simulink model "Es34"  (R2021b)
settings: Solver=FixedStepAuto  StartTime=0.0  StopTime=3  FixedStep=1e-3  RelTol=1e-5
undefined symbols (not defined in the file or in its folder): coriolis, epsilon, gravload, inertia, Kd, Kp, p560, p560_nofric, p560Unc, p560Unc_nf, q_init, rho, Z, Z_1, Z_10
libraries: simulink x5
settings Model: Creator=Andrea  LastModifiedBy=mular
settings SolverCC: AlgebraicLoopSolver=TrustRegion
settings DataIOCC: ReturnWorkspaceOutputs=off
settings DebuggingCC: SFMachineParentedDataDiag=warning  ArithmeticOperatorsInVariantConditions=warning
settings SFSimCC: CustomCodeUndefinedFunction=UseInterfaceOnly

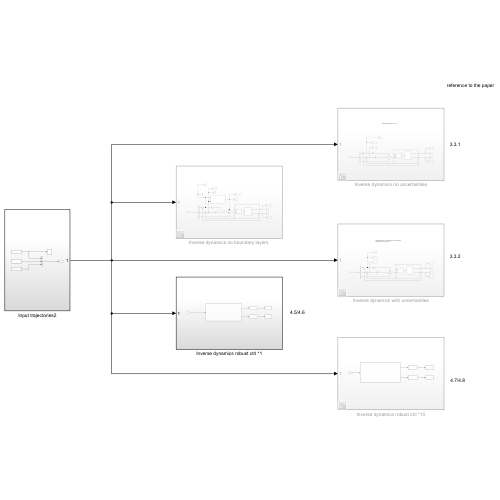
[thumbnail: Simulink's stored preview of the top-level diagram]
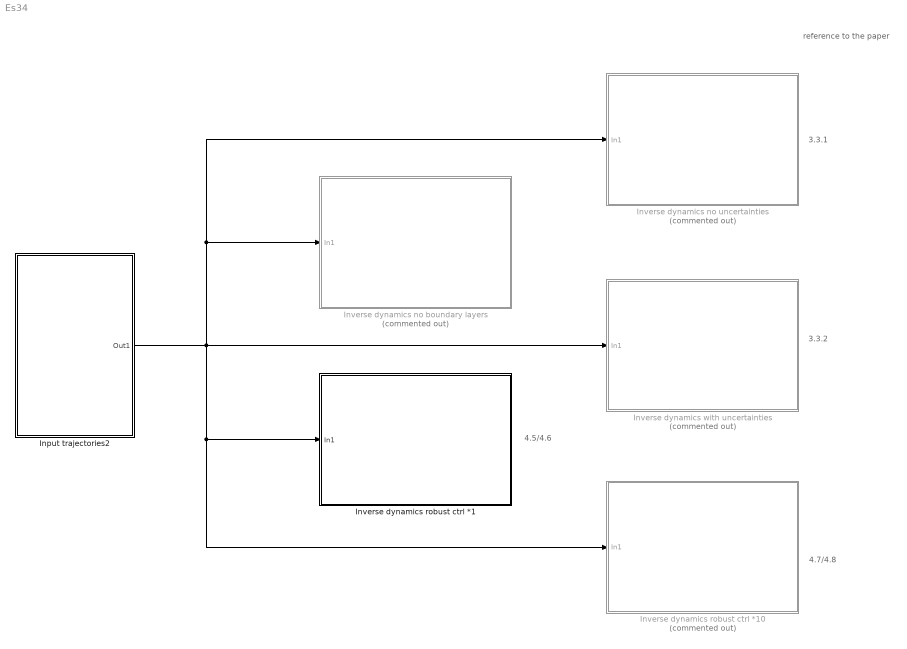
== system Es34 ==
  note: reference to the paper
  note: 4.5/4.6
  note: 4.7/4.8
  note: 3.3.2
  note: 3.3.1
  Input trajectories2 : Subsystem
  "Inverse dynamics no boundary layers " : Subsystem  Commented=on
  Inverse dynamics no uncertainties : Subsystem  Commented=on
  Inverse dynamics robust ctrl *1 : Subsystem
  Inverse dynamics robust ctrl *10 : Subsystem  Commented=on
  Inverse dynamics with uncertainties : Subsystem  Commented=on
  wires:
  Input trajectories2/1(Out1) -> Inverse dynamics no uncertainties/1(In1), "Inverse dynamics no boundary layers "/1(In1), Inverse dynamics robust ctrl *10/1(In1), Inverse dynamics robust ctrl *1/1(In1), Inverse dynamics with uncertainties/1(In1)

== system Es34/Input trajectories2 ==
  From Workspace : FromWorkspace  VariableName=qqs  OutputAfterFinalValue=Holding final value
  From Workspace1 : FromWorkspace  VariableName=qqsd  OutputAfterFinalValue=Holding final value
  From Workspace2 : FromWorkspace  VariableName=qqsdd  OutputAfterFinalValue=Holding final value
  Mux : Mux  Inputs=3
  Scope : Scope
  Out1 : Outport  VectorParamsAs1DForOutWhenUnconnected=off
  wires:
  Mux/1 -> Out1/1
  From Workspace1/1 -> Mux/2
  From Workspace/1 -> Mux/1, Scope/1
  From Workspace2/1 -> Mux/3

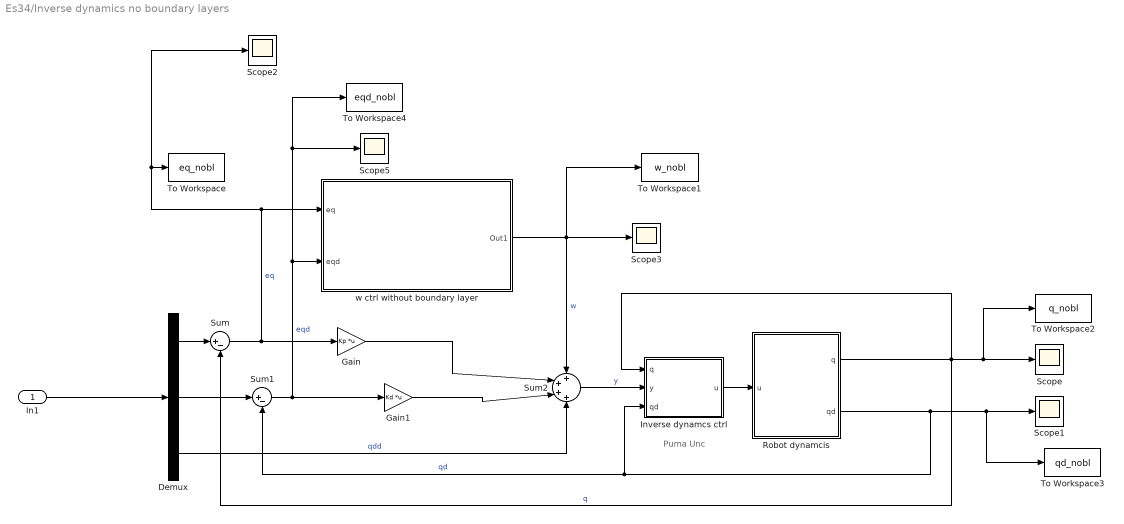
== system Es34/Inverse dynamics no boundary layers  ==
  note: Puma Unc
  In1 : Inport
  Demux : Demux  Outputs=3
  Gain : Gain  Gain=Kp  Multiplication=Matrix(K*u) (u vector)
  Gain1 : Gain  Gain=Kd  Multiplication=Matrix(K*u) (u vector)
  Inverse dynamcs ctrl : Subsystem  mask{mdl=p560Unc}
      mask prompts: mdl "Robot model"
  Robot dynamcis : Subsystem  mask{Realmdl=p560_nofric, q_init=q_init}
      mask prompts: Realmdl "Real robot model"; q_init "Initial position"
  Scope{,1..3,5} (5 alike) : Scope
  Sum : Sum  Inputs=|+-
  Sum1 : Sum  Inputs=|+-
  Sum2 : Sum  Inputs=++++
  To Workspace : ToWorkspace  VariableName=eq_nobl  SampleTime=-1
  To Workspace1 : ToWorkspace  VariableName=w_nobl  SampleTime=-1
  To Workspace2 : ToWorkspace  VariableName=q_nobl  SampleTime=-1
  To Workspace3 : ToWorkspace  VariableName=qd_nobl  SampleTime=-1
  To Workspace4 : ToWorkspace  VariableName=eqd_nobl  SampleTime=-1
  w ctrl without boundary layer : Subsystem
  wires:
  Sum/1 -> Gain/1, w ctrl without boundary layer/1(eq), To Workspace/1, Scope2/1  "eq"
  Sum2/1 -> Inverse dynamcs ctrl/2(y)  "y"
  Sum1/1 -> To Workspace4/1, Scope5/1, w ctrl without boundary layer/2(eqd), Gain1/1  "eqd"
  Demux/2 -> Sum1/1
  Demux/1 -> Sum/1
  Inverse dynamcs ctrl/1(u) -> Robot dynamcis/1(u)
  In1/1 -> Demux/1
  Demux/3 -> Sum2/4  "qdd"
  w ctrl without boundary layer/1(Out1) -> Scope3/1, To Workspace1/1, Sum2/1  "w"
  Robot dynamcis/1(q) -> Inverse dynamcs ctrl/1(q), To Workspace2/1, Scope/1, Sum/2  "q"
  Robot dynamcis/2(qd) -> Scope1/1, To Workspace3/1, Inverse dynamcs ctrl/3(qd), Sum1/2  "qd"
  Gain1/1 -> Sum2/3
  Gain/1 -> Sum2/2

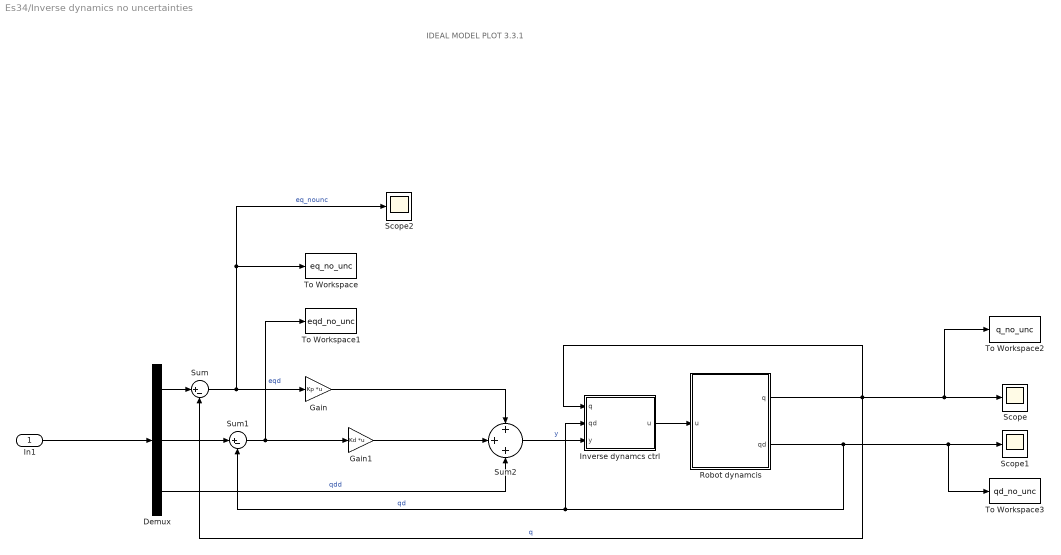
== system Es34/Inverse dynamics no uncertainties ==
  note: IDEAL MODEL PLOT 3.3.1
  In1 : Inport
  Demux : Demux  Outputs=3
  Gain : Gain  Gain=Kp  Multiplication=Matrix(K*u) (u vector)
  Gain1 : Gain  Gain=Kd  Multiplication=Matrix(K*u) (u vector)
  Inverse dynamcs ctrl : Subsystem  mask{mdl=p560Unc_nf}
      mask prompts: mdl "Robot model"
  Robot dynamcis : Subsystem  mask{Realmdl=p560Unc_nf, q_init=q_init}
      mask prompts: Realmdl "Real robot model"; q_init "Initial position"
  Scope : Scope
  Scope1 : Scope
  Scope2 : Scope
  Sum : Sum  Inputs=|+-
  Sum1 : Sum  Inputs=|+-
  Sum2 : Sum  Inputs=+++
  To Workspace : ToWorkspace  VariableName=eq_no_unc  SampleTime=-1
  To Workspace1 : ToWorkspace  VariableName=eqd_no_unc  SampleTime=-1
  To Workspace2 : ToWorkspace  VariableName=q_no_unc  SampleTime=-1
  To Workspace3 : ToWorkspace  VariableName=qd_no_unc  SampleTime=-1
  wires:
  Robot dynamcis/2(qd) -> To Workspace3/1, Scope1/1, Sum1/2, Inverse dynamcs ctrl/2(qd)  "qd"
  Robot dynamcis/1(q) -> Inverse dynamcs ctrl/1(q), To Workspace2/1, Scope/1, Sum/2  "q"
  Gain1/1 -> Sum2/2
  In1/1 -> Demux/1
  Inverse dynamcs ctrl/1(u) -> Robot dynamcis/1(u)
  Demux/1 -> Sum/1
  Demux/2 -> Sum1/1
  Sum1/1 -> To Workspace1/1, Gain1/1  "eqd"
  Sum2/1 -> Inverse dynamcs ctrl/3(y)  "y"
  Sum/1 -> Scope2/1, To Workspace/1, Gain/1  "eq_nounc"
  Gain/1 -> Sum2/1
  Demux/3 -> Sum2/3  "qdd"

== system Es34/Inverse dynamics robust ctrl *1 ==
  In1 : Inport
  Interpreted MATLAB Function1 : MATLABFcn  MATLABFcn=norm(u,2)  OutputDimensions=1
  Interpreted MATLAB Function2 : MATLABFcn  MATLABFcn=norm(u,2)  OutputDimensions=1
  To Workspace : ToWorkspace  VariableName=norm_eq_rc1  SampleTime=-1
  To Workspace1 : ToWorkspace  VariableName=norm_eqd_rc1  SampleTime=-1
  ctrl : Subsystem
  wires:
  In1/1 -> ctrl/1(In1)
  ctrl/1(eq) -> Interpreted MATLAB Function1/1
  Interpreted MATLAB Function1/1 -> To Workspace/1
  Interpreted MATLAB Function2/1 -> To Workspace1/1
  ctrl/2(eqd) -> Interpreted MATLAB Function2/1

== system Es34/Inverse dynamics robust ctrl *10 ==
  In1 : Inport
  Interpreted MATLAB Function1 : MATLABFcn  MATLABFcn=norm(u,2)  OutputDimensions=1
  Interpreted MATLAB Function2 : MATLABFcn  MATLABFcn=norm(u,2)  OutputDimensions=1
  To Workspace : ToWorkspace  VariableName=norm_eq_rc10  SampleTime=-1
  To Workspace1 : ToWorkspace  VariableName=norm_eqd_rc10  SampleTime=-1
  ctrl : Subsystem
  wires:
  ctrl/2(eqd) -> Interpreted MATLAB Function2/1
  Interpreted MATLAB Function2/1 -> To Workspace1/1
  Interpreted MATLAB Function1/1 -> To Workspace/1
  ctrl/1(eq) -> Interpreted MATLAB Function1/1
  In1/1 -> ctrl/1(In1)

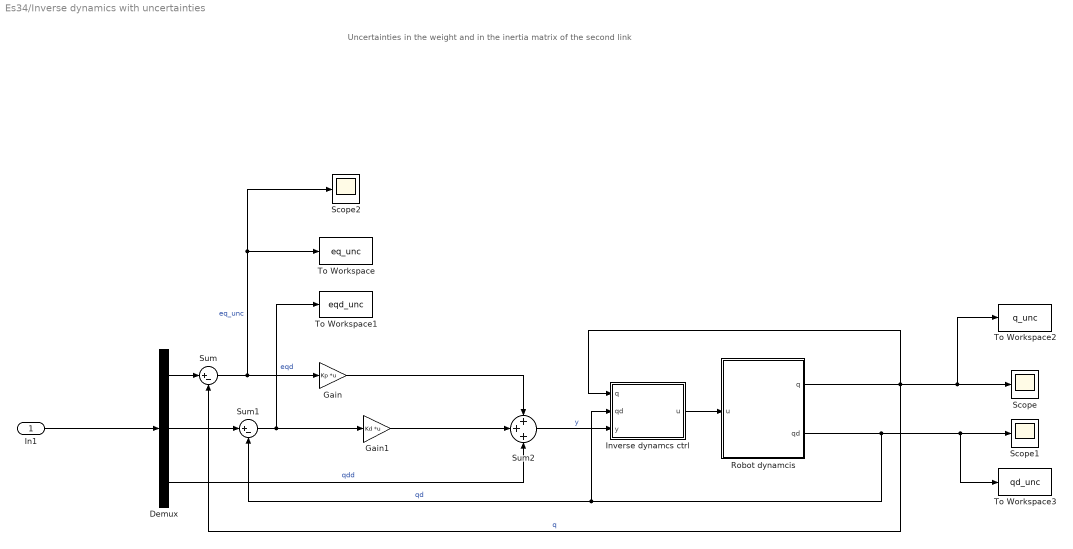
== system Es34/Inverse dynamics with uncertainties ==
  note: Uncertainties in the weight and in the inertia matrix of the second link
  In1 : Inport
  Demux : Demux  Outputs=3
  Gain : Gain  Gain=Kp  Multiplication=Matrix(K*u) (u vector)
  Gain1 : Gain  Gain=Kd  Multiplication=Matrix(K*u) (u vector)
  Inverse dynamcs ctrl : Subsystem  mask{mdl=p560Unc_nf}
      mask prompts: mdl "Robot model"
  Robot dynamcis : Subsystem  mask{Realmdl=p560_nofric, q_init=q_init}
      mask prompts: Realmdl "Real robot model"; q_init "Initial position"
  Scope : Scope
  Scope1 : Scope
  Scope2 : Scope
  Sum : Sum  Inputs=|+-
  Sum1 : Sum  Inputs=|+-
  Sum2 : Sum  Inputs=+++
  To Workspace : ToWorkspace  VariableName=eq_unc  SampleTime=-1
  To Workspace1 : ToWorkspace  VariableName=eqd_unc  SampleTime=-1
  To Workspace2 : ToWorkspace  VariableName=q_unc  SampleTime=-1
  To Workspace3 : ToWorkspace  VariableName=qd_unc  SampleTime=-1
  wires:
  Sum/1 -> Gain/1, Scope2/1, To Workspace/1  "eq_unc"
  Sum2/1 -> Inverse dynamcs ctrl/3(y)  "y"
  Sum1/1 -> To Workspace1/1, Gain1/1  "eqd"
  Demux/2 -> Sum1/1
  Demux/1 -> Sum/1
  Inverse dynamcs ctrl/1(u) -> Robot dynamcis/1(u)
  In1/1 -> Demux/1
  Demux/3 -> Sum2/3  "qdd"
  Gain1/1 -> Sum2/2
  Robot dynamcis/1(q) -> Inverse dynamcs ctrl/1(q), To Workspace2/1, Scope/1, Sum/2  "q"
  Robot dynamcis/2(qd) -> To Workspace3/1, Scope1/1, Inverse dynamcs ctrl/2(qd), Sum1/2  "qd"
  Gain/1 -> Sum2/1

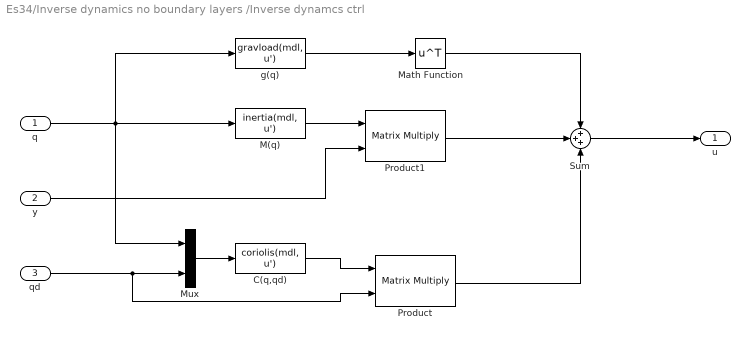
== system Es34/Inverse dynamics no boundary layers /Inverse dynamcs ctrl ==
  q : Inport
  y : Inport  Port=2
  qd : Inport  Port=3
  C(q,qd) : MATLABFcn  MATLABFcn=coriolis(mdl, u')  OutputDimensions=[p560.n p560.n]  Output1D=off
  M(q) : MATLABFcn  MATLABFcn=inertia(mdl, u')  OutputDimensions=[p560.n p560.n]  Output1D=off
  Math Function : Math  Operator=transpose  SignedPower=on  SaturateOnIntegerOverflow=on
  Mux : Mux  Inputs=2
  Product : Product  Multiplication=Matrix(*)
  Product1 : Product  Multiplication=Matrix(*)
  Sum : Sum  Inputs=+++
  g(q) : MATLABFcn  MATLABFcn=gravload(mdl, u')  OutputDimensions=[1 p560.n]  Output1D=off
  u : Outport  VectorParamsAs1DForOutWhenUnconnected=off
  wires:
  q/1 -> M(q)/1, g(q)/1, Mux/1
  Mux/1 -> C(q,qd)/1
  C(q,qd)/1 -> Product/1
  qd/1 -> Product/2, Mux/2
  M(q)/1 -> Product1/1
  y/1 -> Product1/2
  Product1/1 -> Sum/2
  Product/1 -> Sum/3
  Sum/1 -> u/1
  g(q)/1 -> Math Function/1
  Math Function/1 -> Sum/1

== system Es34/Inverse dynamics no boundary layers /Robot dynamcis ==
  u : Inport
  Integrator : Integrator
  Integrator1 : Integrator  InitialCondition=q_init
  Mux : Mux  Inputs=3
  S-Function : S-Function  FunctionName=slaccel  Parameters=Realmdl  SFunctionDeploymentMode=off  EnableBusSupport=off
  q : Outport  VectorParamsAs1DForOutWhenUnconnected=off
  qd : Outport  Port=2  VectorParamsAs1DForOutWhenUnconnected=off
  wires:
  Mux/1 -> S-Function/1
  u/1 -> Mux/3
  Integrator/1 -> qd/1, Mux/2, Integrator1/1  "qd"
  S-Function/1 -> Integrator/1  "qdd"
  Integrator1/1 -> q/1, Mux/1

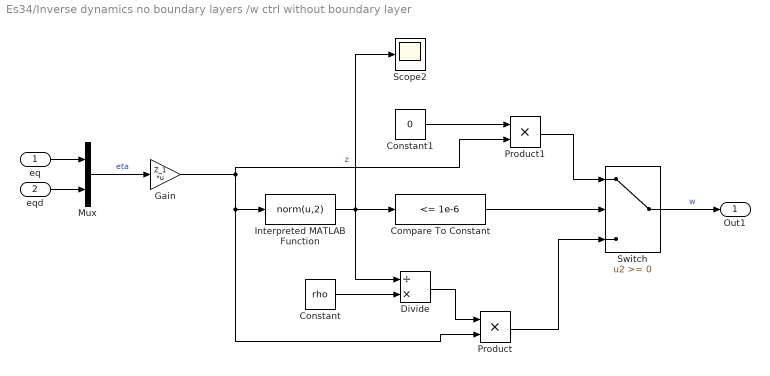
== system Es34/Inverse dynamics no boundary layers /w ctrl without boundary layer ==
  eq : Inport
  eqd : Inport  Port=2
  Compare To Constant : simulink/Logic and Bit Operations/Compare To Constant  relop=<=  const=1e-6  OutDataTypeStr=boolean  ZeroCross=off
  Constant : Constant  Value=rho
  Constant1 : Constant  Value=0
  Divide : Product  Inputs=/*
  Gain : Gain  Gain=Z_1  Multiplication=Matrix(K*u) (u vector)
  Interpreted MATLAB Function : MATLABFcn  MATLABFcn=norm(u,2)
  Mux : Mux  Inputs=2
  Product : Product
  Product1 : Product
  Scope2 : Scope
  Switch : Switch  ZeroCross=off
  Out1 : Outport  VectorParamsAs1DForOutWhenUnconnected=off
  wires:
  eqd/1 -> Mux/2
  Mux/1 -> Gain/1  "eta"
  eq/1 -> Mux/1
  Gain/1 -> Interpreted MATLAB Function/1, Product/2, Product1/2  "z"
  Interpreted MATLAB Function/1 -> Scope2/1, Divide/1, Compare To Constant/1
  Switch/1 -> Out1/1  "w"
  Constant/1 -> Divide/2
  Divide/1 -> Product/1
  Compare To Constant/1 -> Switch/2
  Product/1 -> Switch/3
  Constant1/1 -> Product1/1
  Product1/1 -> Switch/1

== system Es34/Inverse dynamics no uncertainties/Inverse dynamcs ctrl ==
  q : Inport
  qd : Inport  Port=2
  y : Inport  Port=3
  C(q,qd) : MATLABFcn  MATLABFcn=coriolis(mdl, u')  OutputDimensions=[p560.n p560.n]  Output1D=off
  M(q) : MATLABFcn  MATLABFcn=inertia(mdl, u')  OutputDimensions=[p560.n p560.n]  Output1D=off
  Math Function : Math  Operator=transpose  SignedPower=on  SaturateOnIntegerOverflow=on
  Mux : Mux  Inputs=2
  Product : Product  Multiplication=Matrix(*)
  Product1 : Product  Multiplication=Matrix(*)
  Sum : Sum  Inputs=+++
  g(q) : MATLABFcn  MATLABFcn=gravload(mdl, u')  OutputDimensions=[1 p560.n]  Output1D=off
  u : Outport  VectorParamsAs1DForOutWhenUnconnected=off
  wires:
  Math Function/1 -> Sum/1
  g(q)/1 -> Math Function/1
  Sum/1 -> u/1
  Product/1 -> Sum/3
  Product1/1 -> Sum/2
  y/1 -> Product1/2
  M(q)/1 -> Product1/1
  qd/1 -> Mux/2, Product/2
  C(q,qd)/1 -> Product/1
  Mux/1 -> C(q,qd)/1
  q/1 -> Mux/1, M(q)/1, g(q)/1

== system Es34/Inverse dynamics no uncertainties/Robot dynamcis ==
  u : Inport
  Integrator : Integrator
  Integrator1 : Integrator  InitialCondition=q_init
  Mux : Mux  Inputs=3
  S-Function : S-Function  FunctionName=slaccel  Parameters=Realmdl  SFunctionDeploymentMode=off  EnableBusSupport=off
  q : Outport  VectorParamsAs1DForOutWhenUnconnected=off
  qd : Outport  Port=2  VectorParamsAs1DForOutWhenUnconnected=off
  wires:
  Integrator1/1 -> Mux/1, q/1
  S-Function/1 -> Integrator/1  "qdd"
  Integrator/1 -> Integrator1/1, Mux/2, qd/1  "qd"
  u/1 -> Mux/3
  Mux/1 -> S-Function/1

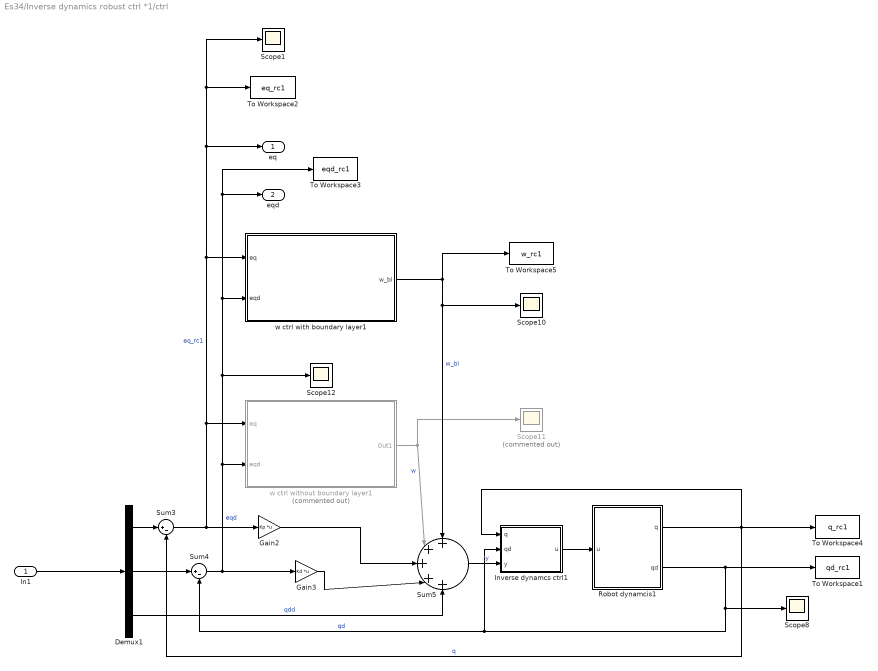
== system Es34/Inverse dynamics robust ctrl *1/ctrl ==
  In1 : Inport
  Demux1 : Demux  Outputs=3
  Gain2 : Gain  Gain=Kp  Multiplication=Matrix(K*u) (u vector)
  Gain3 : Gain  Gain=Kd  Multiplication=Matrix(K*u) (u vector)
  Inverse dynamcs ctrl1 : Subsystem  mask{mdl=p560Unc_nf}
      mask prompts: mdl "Robot model"
  Robot dynamcis1 : Subsystem  mask{Realmdl=p560_nofric, q_init=q_init}
      mask prompts: Realmdl "Real robot model"; q_init "Initial position"
  Scope{1,8,10,12} (4 alike) : Scope
  Scope11 : Scope  Commented=on
  Sum3 : Sum  Inputs=|+-
  Sum4 : Sum  Inputs=|+-
  Sum5 : Sum  Inputs=+++++
  To Workspace1 : ToWorkspace  VariableName=qd_rc1  SampleTime=-1
  To Workspace2 : ToWorkspace  VariableName=eq_rc1  SampleTime=-1
  To Workspace3 : ToWorkspace  VariableName=eqd_rc1  SampleTime=-1
  To Workspace4 : ToWorkspace  VariableName=q_rc1  SampleTime=-1
  To Workspace5 : ToWorkspace  VariableName=w_rc1  SampleTime=-1
  w ctrl with boundary layer1 : Subsystem
  w ctrl without boundary layer1 : Subsystem  Commented=on
  eq : Outport  VectorParamsAs1DForOutWhenUnconnected=off
  eqd : Outport  Port=2  VectorParamsAs1DForOutWhenUnconnected=off
  wires:
  Sum5/1 -> Inverse dynamcs ctrl1/3(y)  "y"
  Robot dynamcis1/1(q) -> Inverse dynamcs ctrl1/1(q), To Workspace4/1, Sum3/2  "q"
  w ctrl without boundary layer1/1(Out1) -> Sum5/2, Scope11/1  "w"
  Sum4/1 -> Scope12/1, eqd/1, To Workspace3/1, w ctrl with boundary layer1/2(eqd), w ctrl without boundary layer1/2(eqd), Gain3/1  "eqd"
  Demux1/2 -> Sum4/1
  Robot dynamcis1/2(qd) -> To Workspace1/1, Inverse dynamcs ctrl1/2(qd), Sum4/2, Scope8/1  "qd"
  Sum3/1 -> w ctrl with boundary layer1/1(eq), To Workspace2/1, Scope1/1, eq/1, w ctrl without boundary layer1/1(eq), Gain2/1  "eq_rc1"
  In1/1 -> Demux1/1
  Inverse dynamcs ctrl1/1(u) -> Robot dynamcis1/1(u)
  Demux1/1 -> Sum3/1
  Demux1/3 -> Sum5/5  "qdd"
  Gain2/1 -> Sum5/3
  w ctrl with boundary layer1/1(w_bl) -> To Workspace5/1, Sum5/1, Scope10/1  "w_bl"
  Gain3/1 -> Sum5/4

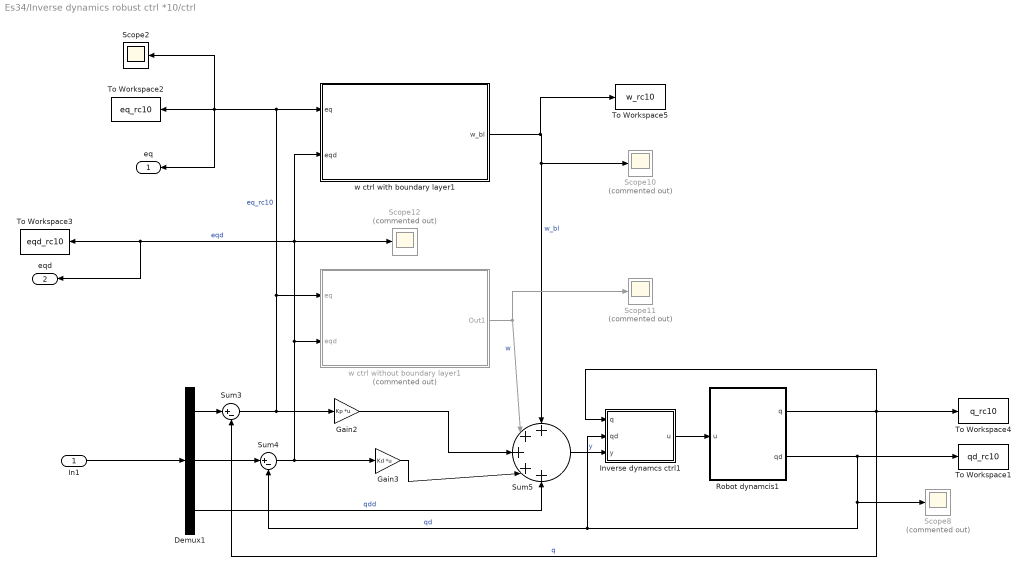
== system Es34/Inverse dynamics robust ctrl *10/ctrl ==
  In1 : Inport
  Demux1 : Demux  Outputs=3
  Gain2 : Gain  Gain=Kp  Multiplication=Matrix(K*u) (u vector)
  Gain3 : Gain  Gain=Kd  Multiplication=Matrix(K*u) (u vector)
  Inverse dynamcs ctrl1 : Subsystem  mask{mdl=p560Unc_nf}
      mask prompts: mdl "Robot model"
  Robot dynamcis1 : Subsystem  mask{Realmdl=p560_nofric, q_init=q_init}
      mask prompts: Realmdl "Real robot model"; q_init "Initial position"
  Scope{8,10..12} (4 alike) : Scope  Commented=on
  Scope2 : Scope
  Sum3 : Sum  Inputs=|+-
  Sum4 : Sum  Inputs=|+-
  Sum5 : Sum  Inputs=+++++
  To Workspace1 : ToWorkspace  VariableName=qd_rc10  SampleTime=-1
  To Workspace2 : ToWorkspace  VariableName=eq_rc10  SampleTime=-1
  To Workspace3 : ToWorkspace  VariableName=eqd_rc10  SampleTime=-1
  To Workspace4 : ToWorkspace  VariableName=q_rc10  SampleTime=-1
  To Workspace5 : ToWorkspace  VariableName=w_rc10  SampleTime=-1
  w ctrl with boundary layer1 : Subsystem
  w ctrl without boundary layer1 : Subsystem  Commented=on
  eq : Outport  VectorParamsAs1DForOutWhenUnconnected=off
  eqd : Outport  Port=2  VectorParamsAs1DForOutWhenUnconnected=off
  wires:
  Gain3/1 -> Sum5/4
  w ctrl with boundary layer1/1(w_bl) -> To Workspace5/1, Scope10/1, Sum5/1  "w_bl"
  Gain2/1 -> Sum5/3
  Demux1/3 -> Sum5/5  "qdd"
  Demux1/1 -> Sum3/1
  Inverse dynamcs ctrl1/1(u) -> Robot dynamcis1/1(u)
  In1/1 -> Demux1/1
  Sum3/1 -> Gain2/1, w ctrl without boundary layer1/1(eq), Scope2/1, To Workspace2/1, eq/1, w ctrl with boundary layer1/1(eq)  "eq_rc10"
  Robot dynamcis1/2(qd) -> Scope8/1, Sum4/2, Inverse dynamcs ctrl1/2(qd), To Workspace1/1  "qd"
  Demux1/2 -> Sum4/1
  Sum4/1 -> Gain3/1, w ctrl without boundary layer1/2(eqd), w ctrl with boundary layer1/2(eqd), eqd/1, To Workspace3/1, Scope12/1  "eqd"
  w ctrl without boundary layer1/1(Out1) -> Scope11/1, Sum5/2  "w"
  Robot dynamcis1/1(q) -> Sum3/2, To Workspace4/1, Inverse dynamcs ctrl1/1(q)  "q"
  Sum5/1 -> Inverse dynamcs ctrl1/3(y)  "y"

== system Es34/Inverse dynamics with uncertainties/Inverse dynamcs ctrl ==
  q : Inport
  qd : Inport  Port=2
  y : Inport  Port=3
  C(q,qd) : MATLABFcn  MATLABFcn=coriolis(mdl, u')  OutputDimensions=[p560.n p560.n]  Output1D=off
  M(q) : MATLABFcn  MATLABFcn=inertia(mdl, u')  OutputDimensions=[p560.n p560.n]  Output1D=off
  Math Function : Math  Operator=transpose  SignedPower=on  SaturateOnIntegerOverflow=on
  Mux : Mux  Inputs=2
  Product : Product  Multiplication=Matrix(*)
  Product1 : Product  Multiplication=Matrix(*)
  Sum : Sum  Inputs=+++
  g(q) : MATLABFcn  MATLABFcn=gravload(mdl, u')  OutputDimensions=[1 p560.n]  Output1D=off
  u : Outport  VectorParamsAs1DForOutWhenUnconnected=off
  wires:
  q/1 -> M(q)/1, Mux/1, g(q)/1
  Mux/1 -> C(q,qd)/1
  C(q,qd)/1 -> Product/1
  qd/1 -> Product/2, Mux/2
  M(q)/1 -> Product1/1
  y/1 -> Product1/2
  Product1/1 -> Sum/2
  Product/1 -> Sum/3
  Sum/1 -> u/1
  g(q)/1 -> Math Function/1
  Math Function/1 -> Sum/1

== system Es34/Inverse dynamics with uncertainties/Robot dynamcis ==
  u : Inport
  Integrator : Integrator
  Integrator1 : Integrator  InitialCondition=q_init
  Mux : Mux  Inputs=3
  S-Function : S-Function  FunctionName=slaccel  Parameters=Realmdl  SFunctionDeploymentMode=off  EnableBusSupport=off
  q : Outport  VectorParamsAs1DForOutWhenUnconnected=off
  qd : Outport  Port=2  VectorParamsAs1DForOutWhenUnconnected=off
  wires:
  Mux/1 -> S-Function/1
  u/1 -> Mux/3
  Integrator/1 -> qd/1, Mux/2, Integrator1/1  "qd"
  S-Function/1 -> Integrator/1  "qdd"
  Integrator1/1 -> q/1, Mux/1

== system Es34/Inverse dynamics robust ctrl *1/ctrl/Inverse dynamcs ctrl1 ==
  q : Inport
  qd : Inport  Port=2
  y : Inport  Port=3
  C(q,qd) : MATLABFcn  MATLABFcn=coriolis(mdl, u')  OutputDimensions=[p560.n p560.n]  Output1D=off
  M(q) : MATLABFcn  MATLABFcn=inertia(mdl, u')  OutputDimensions=[p560.n p560.n]  Output1D=off
  Math Function : Math  Operator=transpose  SignedPower=on  SaturateOnIntegerOverflow=on
  Mux : Mux  Inputs=2
  Product : Product  Multiplication=Matrix(*)
  Product1 : Product  Multiplication=Matrix(*)
  Sum : Sum  Inputs=+++
  g(q) : MATLABFcn  MATLABFcn=gravload(mdl, u')  OutputDimensions=[1 p560.n]  Output1D=off
  u : Outport  VectorParamsAs1DForOutWhenUnconnected=off
  wires:
  q/1 -> M(q)/1, g(q)/1, Mux/1
  Mux/1 -> C(q,qd)/1
  C(q,qd)/1 -> Product/1
  qd/1 -> Product/2, Mux/2
  M(q)/1 -> Product1/1
  y/1 -> Product1/2
  Product1/1 -> Sum/2
  Product/1 -> Sum/3
  Sum/1 -> u/1
  g(q)/1 -> Math Function/1
  Math Function/1 -> Sum/1

== system Es34/Inverse dynamics robust ctrl *1/ctrl/Robot dynamcis1 ==
  u : Inport
  Integrator : Integrator
  Integrator1 : Integrator  InitialCondition=q_init
  Mux : Mux  Inputs=3
  S-Function : S-Function  FunctionName=slaccel  Parameters=Realmdl  SFunctionDeploymentMode=off  EnableBusSupport=off
  q : Outport  VectorParamsAs1DForOutWhenUnconnected=off
  qd : Outport  Port=2  VectorParamsAs1DForOutWhenUnconnected=off
  wires:
  Mux/1 -> S-Function/1
  u/1 -> Mux/3
  Integrator/1 -> qd/1, Mux/2, Integrator1/1  "qd"
  S-Function/1 -> Integrator/1  "qdd"
  Integrator1/1 -> q/1, Mux/1

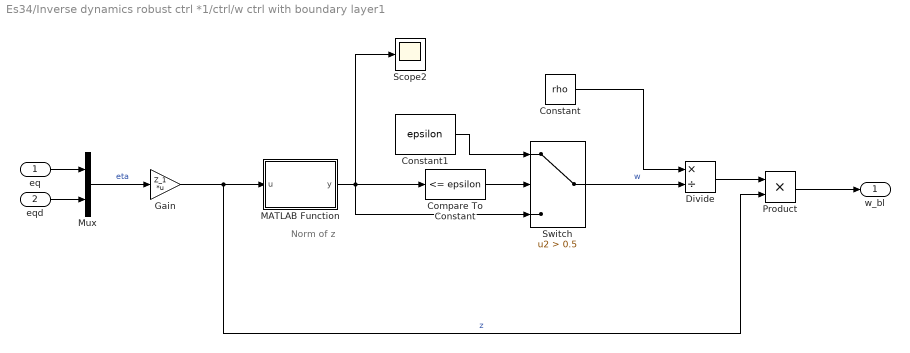
== system Es34/Inverse dynamics robust ctrl *1/ctrl/w ctrl with boundary layer1 ==
  note: Norm of z
  eq : Inport
  eqd : Inport  Port=2
  Compare To Constant : simulink/Logic and Bit Operations/Compare To Constant  relop=<=  const=epsilon  OutDataTypeStr=boolean
  Constant : Constant  Value=rho
  Constant1 : Constant  Value=epsilon
  Divide : Product  Inputs=*/
  Gain : Gain  Gain=Z_1  Multiplication=Matrix(K*u) (u vector)
  MATLAB Function : MATLAB Function  TreatAsAtomicUnit=on
  Mux : Mux  Inputs=2
  Product : Product
  Scope2 : Scope
  Switch : Switch  Criteria=u2 > Threshold  Threshold=0.5  ZeroCross=off
  w_bl : Outport  VectorParamsAs1DForOutWhenUnconnected=off
  wires:
  MATLAB Function/1(y) -> Switch/3, Compare To Constant/1, Scope2/1
  Gain/1 -> Product/2, MATLAB Function/1(u)  "z"
  eq/1 -> Mux/1
  Mux/1 -> Gain/1  "eta"
  eqd/1 -> Mux/2
  Compare To Constant/1 -> Switch/2
  Constant/1 -> Divide/1
  Switch/1 -> Divide/2  "w"
  Divide/1 -> Product/1
  Product/1 -> w_bl/1
  Constant1/1 -> Switch/1

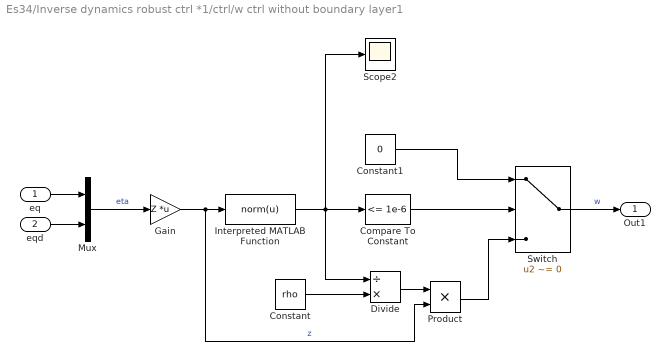
== system Es34/Inverse dynamics robust ctrl *1/ctrl/w ctrl without boundary layer1 ==
  eq : Inport
  eqd : Inport  Port=2
  Compare To Constant : simulink/Logic and Bit Operations/Compare To Constant  relop=<=  const=1e-6  OutDataTypeStr=boolean  ZeroCross=off
  Constant : Constant  Value=rho
  Constant1 : Constant  Value=0
  Divide : Product  Inputs=/*
  Gain : Gain  Gain=Z  Multiplication=Matrix(K*u) (u vector)
  Interpreted MATLAB Function : MATLABFcn  MATLABFcn=norm(u)
  Mux : Mux  Inputs=2
  Product : Product
  Scope2 : Scope
  Switch : Switch  Criteria=u2 ~= 0  ZeroCross=off
  Out1 : Outport  VectorParamsAs1DForOutWhenUnconnected=off
  wires:
  eqd/1 -> Mux/2
  Mux/1 -> Gain/1  "eta"
  eq/1 -> Mux/1
  Gain/1 -> Product/2, Interpreted MATLAB Function/1  "z"
  Interpreted MATLAB Function/1 -> Scope2/1, Divide/1, Compare To Constant/1
  Switch/1 -> Out1/1  "w"
  Constant/1 -> Divide/2
  Divide/1 -> Product/1
  Compare To Constant/1 -> Switch/2
  Constant1/1 -> Switch/1
  Product/1 -> Switch/3

== system Es34/Inverse dynamics robust ctrl *10/ctrl/Inverse dynamcs ctrl1 ==
  q : Inport
  qd : Inport  Port=2
  y : Inport  Port=3
  C(q,qd) : MATLABFcn  MATLABFcn=coriolis(mdl, u')  OutputDimensions=[p560.n p560.n]  Output1D=off
  M(q) : MATLABFcn  MATLABFcn=inertia(mdl, u')  OutputDimensions=[p560.n p560.n]  Output1D=off
  Math Function : Math  Operator=transpose  SignedPower=on  SaturateOnIntegerOverflow=on
  Mux : Mux  Inputs=2
  Product : Product  Multiplication=Matrix(*)
  Product1 : Product  Multiplication=Matrix(*)
  Sum : Sum  Inputs=+++
  g(q) : MATLABFcn  MATLABFcn=gravload(mdl, u')  OutputDimensions=[1 p560.n]  Output1D=off
  u : Outport  VectorParamsAs1DForOutWhenUnconnected=off
  wires:
  Math Function/1 -> Sum/1
  g(q)/1 -> Math Function/1
  Sum/1 -> u/1
  Product/1 -> Sum/3
  Product1/1 -> Sum/2
  y/1 -> Product1/2
  M(q)/1 -> Product1/1
  qd/1 -> Mux/2, Product/2
  C(q,qd)/1 -> Product/1
  Mux/1 -> C(q,qd)/1
  q/1 -> Mux/1, g(q)/1, M(q)/1

== system Es34/Inverse dynamics robust ctrl *10/ctrl/Robot dynamcis1 ==
  u : Inport
  Integrator : Integrator
  Integrator1 : Integrator  InitialCondition=q_init
  Mux : Mux  Inputs=3
  S-Function : S-Function  FunctionName=slaccel  Parameters=Realmdl  SFunctionDeploymentMode=off  EnableBusSupport=off
  q : Outport  VectorParamsAs1DForOutWhenUnconnected=off
  qd : Outport  Port=2  VectorParamsAs1DForOutWhenUnconnected=off
  wires:
  Integrator1/1 -> Mux/1, q/1
  S-Function/1 -> Integrator/1  "qdd"
  Integrator/1 -> Integrator1/1, Mux/2, qd/1  "qd"
  u/1 -> Mux/3
  Mux/1 -> S-Function/1

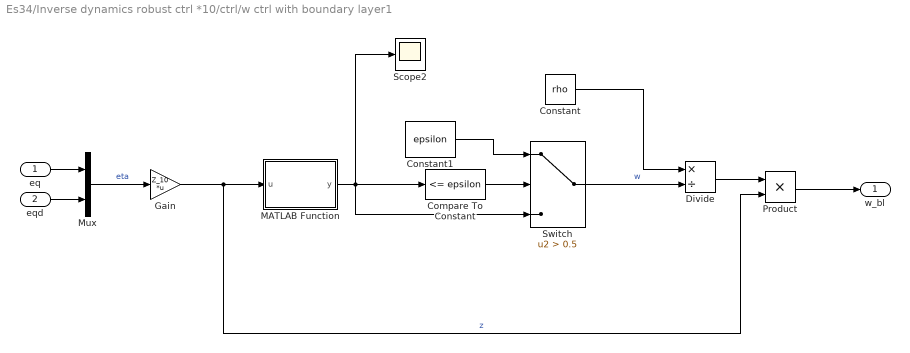
== system Es34/Inverse dynamics robust ctrl *10/ctrl/w ctrl with boundary layer1 ==
  eq : Inport
  eqd : Inport  Port=2
  Compare To Constant : simulink/Logic and Bit Operations/Compare To Constant  relop=<=  const=epsilon  OutDataTypeStr=boolean
  Constant : Constant  Value=rho
  Constant1 : Constant  Value=epsilon
  Divide : Product  Inputs=*/
  Gain : Gain  Gain=Z_10  Multiplication=Matrix(K*u) (u vector)
  MATLAB Function : MATLAB Function  TreatAsAtomicUnit=on
  Mux : Mux  Inputs=2
  Product : Product
  Scope2 : Scope
  Switch : Switch  Criteria=u2 > Threshold  Threshold=0.5  ZeroCross=off
  w_bl : Outport  VectorParamsAs1DForOutWhenUnconnected=off
  wires:
  Constant1/1 -> Switch/1
  Product/1 -> w_bl/1
  Divide/1 -> Product/1
  Switch/1 -> Divide/2  "w"
  Constant/1 -> Divide/1
  Compare To Constant/1 -> Switch/2
  eqd/1 -> Mux/2
  Mux/1 -> Gain/1  "eta"
  eq/1 -> Mux/1
  Gain/1 -> MATLAB Function/1(u), Product/2  "z"
  MATLAB Function/1(y) -> Scope2/1, Compare To Constant/1, Switch/3

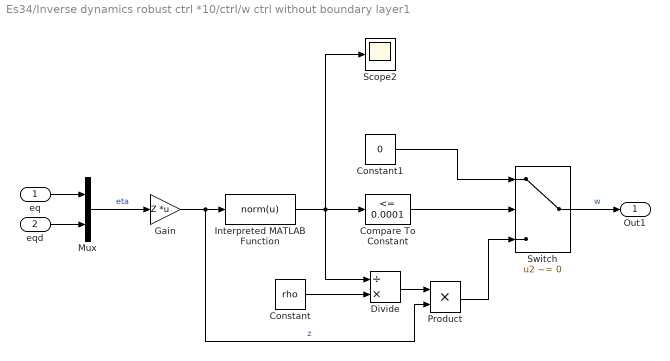
== system Es34/Inverse dynamics robust ctrl *10/ctrl/w ctrl without boundary layer1 ==
  eq : Inport
  eqd : Inport  Port=2
  Compare To Constant : simulink/Logic and Bit Operations/Compare To Constant  relop=<=  const=0.0001  OutDataTypeStr=boolean  ZeroCross=off
  Constant : Constant  Value=rho
  Constant1 : Constant  Value=0
  Divide : Product  Inputs=/*
  Gain : Gain  Gain=Z  Multiplication=Matrix(K*u) (u vector)
  Interpreted MATLAB Function : MATLABFcn  MATLABFcn=norm(u)
  Mux : Mux  Inputs=2
  Product : Product
  Scope2 : Scope
  Switch : Switch  Criteria=u2 ~= 0  ZeroCross=off
  Out1 : Outport  VectorParamsAs1DForOutWhenUnconnected=off
  wires:
  Product/1 -> Switch/3
  Constant1/1 -> Switch/1
  Compare To Constant/1 -> Switch/2
  Divide/1 -> Product/1
  Constant/1 -> Divide/2
  Switch/1 -> Out1/1  "w"
  Interpreted MATLAB Function/1 -> Compare To Constant/1, Divide/1, Scope2/1
  Gain/1 -> Interpreted MATLAB Function/1, Product/2  "z"
  eq/1 -> Mux/1
  Mux/1 -> Gain/1  "eta"
  eqd/1 -> Mux/2

== matlab function Es34/Inverse dynamics robust ctrl *10/ctrl/w ctrl with boundary layer1/MATLAB Function ==
  data: u input; y output
function y = fcn(u)
y = norm(u);

== matlab function Es34/Inverse dynamics robust ctrl *1/ctrl/w ctrl with boundary layer1/MATLAB Function ==
  data: u input; y output
function y = fcn(u)
y = norm(u);
